simulink model "ADP_USB"  (R2017a)
settings: Solver=ode1  StartTime=0.0  StopTime=30  FixedStep=tau  RelTol=1e-3  EnableMultiTasking=on
InitFcn:
  | ADP_USB_Init
undefined symbols (not defined in the file or in its folder): K, T, tau, wcInit
libraries: simulink x4, simulink_extras x4, quanser_aero x1, quarc_library x1
settings Model: SimulationMode=external  ExtModeTrigDuration=10000  Creator=gjaniak  LastModifiedBy=gjaniak
settings SolverCC: PositivePriorityOrder=on
settings DataIOCC: SaveFormat=Array
settings DebuggingCC: SolverPrmCheckMsg=warning  SFUnexpectedBacktrackingDiag=warning  SFNoUnconditionalDefaultTransitionDiag=warning  SFExecutionAtInitializationDiag=none
settings ModelReferenceCC: PropagateSignalLabelsOutOfModel=off
settings RTWCC: SystemTargetFile=quarc_win64.tlc  TemplateMakefile=quarc_default_tmf  Description=QUARC Win64 Target
settings STFCustomTargetCC: TargetPreCompLibLocation=C:\PROGRA~3\QUARC\lib\2017a\win64\release  TargetLangStandard=C99 (ISO)  ConcurrentExecutionCompliant=on  SystemTargetFile=quarc_win64.tlc
settings GRTTargetCC: TargetPreCompLibLocation=C:\PROGRA~3\QUARC\lib\2017a\win64\release  ParMdlRefBuildCompliant=off  CompOptLevelCompliant=off  CombineOutputUpdateFcns=off  MatFileLogging=off  CPPClassGenCompliant=off  GRTInterface=on  UseToolchainInfoCompliant=off  ExtMode=on  ExtModeMexFile=quarc_comm

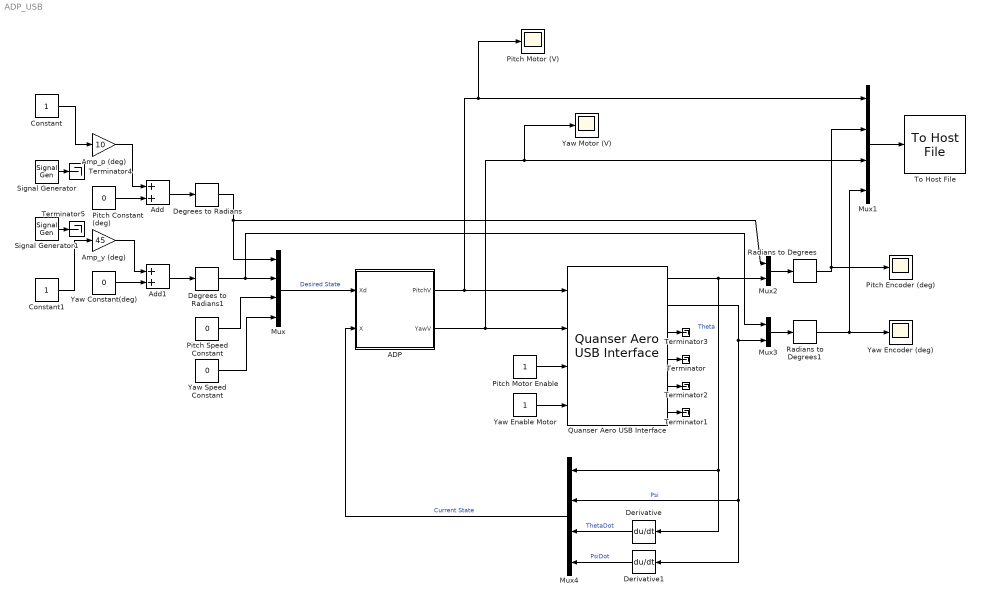
== system ADP_USB ==
  ADP : Subsystem
  Add : Sum
  Add1 : Sum
  Amp_p (deg) : Gain  Gain=10
  Amp_y (deg) : Gain  Gain=45
  Constant : Constant
  Constant1 : Constant
  Degrees to Radians : simulink_extras/Transformations/Degrees to Radians
  Degrees to Radians1 : simulink_extras/Transformations/Degrees to Radians
  Derivative : Derivative
  Derivative1 : Derivative
  Mux : Mux
  Mux1 : Mux
  Mux2 : Mux  Inputs=2
  Mux3 : Mux  Inputs=2
  Mux4 : Mux
  Pitch Constant (deg) : Constant  Value=0
  Pitch Encoder (deg) : Scope
  Pitch Motor (V) : Scope
  Pitch Motor Enable : Constant
  Pitch Speed Constant : Constant  Value=0
  Quanser Aero USB Interface : quanser_aero/Quanser Aero USB Interface
  Radians to Degrees : simulink_extras/Transformations/Radians to Degrees
  Radians to Degrees1 : simulink_extras/Transformations/Radians to Degrees
  Signal Generator : SignalGenerator  WaveForm=square  Frequency=0.1
  Signal Generator1 : SignalGenerator  WaveForm=square  Frequency=0.04
  Terminator{,1..5} (6 alike) : Terminator
  To Host File : quarc_library/Sinks/To Host/To Host File  file_name=ADP_USB_Square.mat  variable_name=ADP_USB_Square  decimation=1  sample_time=-1  file_format=MAT-file v.4  options=No header or footer  append=off  final_file_name=ADP_USB_Square.mat  bitrate=2000000
  Yaw Constant(deg) : Constant  Value=0
  Yaw Enable Motor : Constant
  Yaw Encoder (deg) : Scope
  Yaw Motor (V) : Scope
  Yaw Speed Constant : Constant  Value=0
  wires:
  Yaw Enable Motor/1 -> Quanser Aero USB Interface/4
  Pitch Motor Enable/1 -> Quanser Aero USB Interface/3
  Quanser Aero USB Interface/4 -> Terminator/1
  Quanser Aero USB Interface/6 -> Terminator1/1
  Quanser Aero USB Interface/5 -> Terminator2/1
  Quanser Aero USB Interface/3 -> Terminator3/1
  Pitch Constant (deg)/1 -> Add/2
  Add1/1 -> Degrees to Radians1/1
  Amp_p (deg)/1 -> Add/1
  Yaw Constant(deg)/1 -> Add1/2
  Add/1 -> Degrees to Radians/1
  Amp_y (deg)/1 -> Add1/1
  Degrees to Radians/1 -> Mux2/1, Mux/1
  Degrees to Radians1/1 -> Mux3/1, Mux/2
  Pitch Speed Constant/1 -> Mux/3
  Yaw Speed Constant/1 -> Mux/4
  Quanser Aero USB Interface/1 -> Derivative/1, Mux4/1, Mux2/2  "Theta"
  Quanser Aero USB Interface/2 -> Derivative1/1, Mux4/2, Mux3/2  "Psi"
  Mux/1 -> ADP/1(Xd)  "Desired State"
  Mux1/1 -> To Host File/1
  ADP/1(PitchV) -> Pitch Motor (V)/1, Mux1/1, Quanser Aero USB Interface/1
  ADP/2(YawV) -> Yaw Motor (V)/1, Mux1/3, Quanser Aero USB Interface/2
  Mux3/1 -> Radians to Degrees1/1
  Mux2/1 -> Radians to Degrees/1
  Radians to Degrees/1 -> Pitch Encoder (deg)/1, Mux1/2
  Radians to Degrees1/1 -> Yaw Encoder (deg)/1, Mux1/4
  Derivative/1 -> Mux4/3  "ThetaDot"
  Derivative1/1 -> Mux4/4  "PsiDot"
  Mux4/1 -> ADP/2(X)  "Current State"
  Signal Generator/1 -> Terminator4/1
  Constant/1 -> Amp_p (deg)/1
  Signal Generator1/1 -> Terminator5/1
  Constant1/1 -> Amp_y (deg)/1

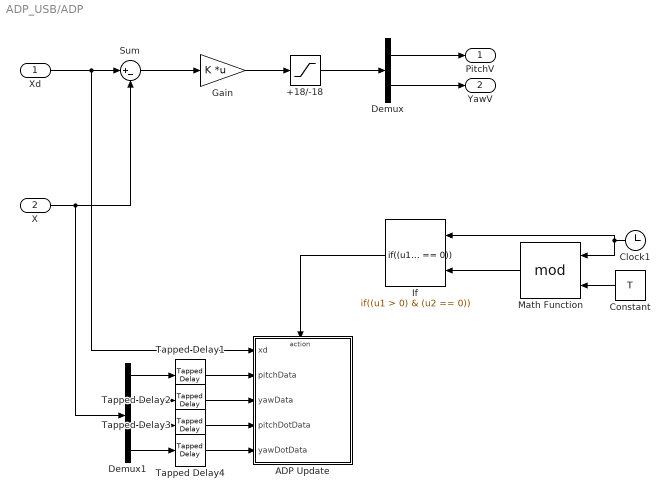
== system ADP_USB/ADP ==
  Xd : Inport
  X : Inport  Port=2
  +18/-18 : Saturate  UpperLimit=18  LowerLimit=-18
  ADP Update : Subsystem  TreatAsAtomicUnit=on
  Clock1 : Clock
  Constant : Constant  Value=T
  Demux : Demux  Outputs=2
  Demux1 : Demux
  Gain : Gain  Gain=K  Multiplication=Matrix(K*u)
  If : If  NumInputs=2  IfExpression=(u1 > 0) & (u2 == 0)  ShowElse=off
  Math Function : Math  Operator=mod  SaturateOnIntegerOverflow=on
  Sum : Sum  Inputs=|+-
  Tapped Delay{1..4} (4 alike) : simulink/Discrete/Tapped Delay  vinit=0.0  samptime=-1  NumDelays=floor(T/tau)  DelayOrder=Oldest  includeCurrent=off
  PitchV : Outport
  YawV : Outport  Port=2
  wires:
  Xd/1 -> ADP Update/1(xd), Sum/1
  Sum/1 -> Gain/1
  Gain/1 -> +18/-18/1
  +18/-18/1 -> Demux/1
  Demux/1 -> PitchV/1
  Demux/2 -> YawV/1
  If/1 -> ADP Update/Action
  Math Function/1 -> If/2
  Constant/1 -> Math Function/2
  Clock1/1 -> If/1, Math Function/1
  X/1 -> Demux1/1, Sum/2
  Demux1/1 -> Tapped Delay1/1
  Tapped Delay1/1 -> ADP Update/2(pitchData)
  Demux1/2 -> Tapped Delay2/1
  Tapped Delay2/1 -> ADP Update/3(yawData)
  Demux1/3 -> Tapped Delay3/1
  Tapped Delay3/1 -> ADP Update/4(pitchDotData)
  Demux1/4 -> Tapped Delay4/1
  Tapped Delay4/1 -> ADP Update/5(yawDotData)

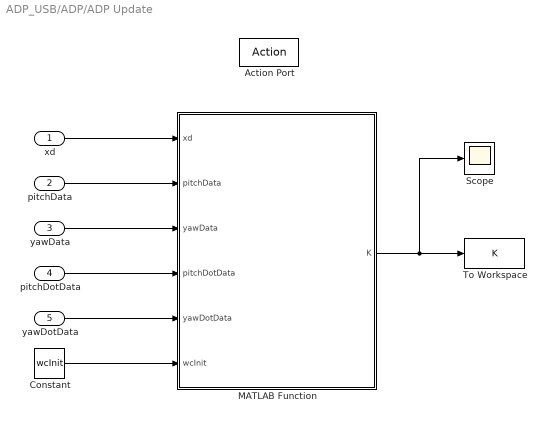
== system ADP_USB/ADP/ADP Update ==
  xd : Inport
  pitchData : Inport  Port=2
  yawData : Inport  Port=3
  pitchDotData : Inport  Port=4
  yawDotData : Inport  Port=5
  Action Port : ActionPort  ActionType=then
  Constant : Constant  Value=wcInit
  MATLAB Function : MATLAB Function  TreatAsAtomicUnit=on
  Scope : Scope
  To Workspace : ToWorkspace  VariableName=K  SampleTime=-1
  wires:
  MATLAB Function/1(K) -> Scope/1, To Workspace/1
  yawData/1 -> MATLAB Function/3(yawData)
  pitchDotData/1 -> MATLAB Function/4(pitchDotData)
  yawDotData/1 -> MATLAB Function/5(yawDotData)
  pitchData/1 -> MATLAB Function/2(pitchData)
  xd/1 -> MATLAB Function/1(xd)
  Constant/1 -> MATLAB Function/6(wcInit)

== matlab function ADP_USB/ADP/ADP Update/MATLAB Function ==
  data: xd input; pitchData input; yawData input; pitchDotData input; yawDotData input; K output; wcInit input
% CRITIC WEIGHT TUNING NEURAL NETWORK
% This function is specific to the helicopter because of the number of
% weights and error model
% THIS FUNCTION CANNOT HAVE ANY ANONYMOUS FUNCTIONS DUE TO THE C CODE
% GENERATION UNSUPPORTING IT
function K = quanserAEROCriticTuning(xd,pitchData,yawData,pitchDotData,yawDotData,wcInit)
    % CREATE THE ERROR VECTOR MATRIX
    % Use the data from the tapped delay blocks to create the error state
    % vector matrix
    e_vec = [pitchData'; yawData'; pitchDotData'; yawDotData'];
    
    % REFERENCE DR. MIAH'S PAPER FOR EQUATION NUMBERS
    % Sampling time [s]
    tau = 0.05;
    
    % COST FUNCTION
    % Q and R matrices used in the cost function
    Q_Mat = diag([270 100 1 1]);
    R_Mat = 0.005*diag([1 1]);
    
    % SYSTEM PARAMETERS SPECIFIC TO THE 2-DOF QUANSER AERO
    A = [0 0 1 0; 0 0 0 1; -1.7442 0 -0.3307 0; 0 0 0 -0.9283];
    B = [0 0; 0 0; -0.0149 0.0414; -0.0751 -0.1295];
    % UNCOMMENT TO USE A STATE-SPACE MODEL THAT IS NOT THE CORRECT ONE DERIVED
    % A = [1 1 1 1; 1 1 1 1; 1 1 1 1; 1 1 1 1];
    % B = [0 0; 0 0; 0.1 0.1; -0.3 -0.3];
    % System dimensions specific for our model
    [n,~] = size(B);
    
    % ERROR MODEL OF THE HELICOPTER
    % gbar and hbar -- EQ 8
    % An anonymous function cannot be used for fbar
    gbar = -B;
    hbar = -A*xd;
    
    % DISCRETE-TIME ERROR MODEL FOR TIME TAU
    % g and h -- EQ 10
    % An anonymous function cannot be used for f
    g = gbar*tau;
    h = hbar*tau;
    
    % COST FUNCTION PARAMETERS
    % The Q matrix cannot be treated as an anonymous function as in the
    % MATLAB simulations
    % Control penalizing matrix in the continuous cost function
    Rbar = R_Mat;
    % The discrete-time cost function will have terms:
    % Right after EQ 11 in paper
    % Control penalizing matrix in the discretized cost function
    R = Rbar*tau;
    
    % NEURAL NETWORK FUNCTIONS
    % These functions cannot be written as anonymous functions as in the
    % MATLAB simulations
    
    % TOLERANCES
    % Convergence tolerance for control policy 
    EpsilonPolicy = 0.1;
    % Convergence tolerance for critic neural network
    EpsilonWcritic = 0.1;
    
    % TRAINING PARAMETERS
    % Number of outer loop iterations
    outerLoopMax = 700;
    % Number of inner loop iterations
    innerLoopMax = 100;
    % Number of equations needed for training, number of sub-intervals
    % Number of training samples
    [~,nbar] = size(e_vec);

    % WEIGHT INITIALIZATION
    % Initialize the weights of the critic neural network to zero
    % Number of rows hard-coded for the helicopter
    WcLast = zeros(14,1);
    
    % LEAST-SQUARES COMPUTATION INITIALIZATION
    % Matrices required for computing least squares weights of the critic 
    % neural networks -- EQ 20
    V = zeros(nbar,1);
    Lambda = zeros(nbar,14);
    
    % Matrix to hold the derivative of the error model during policy
    % updating
    e_k_plus_1 = zeros(n,nbar);
    
    % Product of the least squares matrices must be invertible
    % Logic flag indicating if the critic weights are unsolvable
    % The weights are unsolvable because the least squares matrices have no
    % solution -- not invertible
    diverged = 0;
    
    % OUTER LOOP
    for i = 1:(outerLoopMax-1)
    % Determine if the least squares matrices are invertible
    if diverged == 0
        % For each of the data collection (discrete time index)
        for k = 1:nbar
            % Initialize the optimal inputs to zero 
            uNew = [0; 0];
            % INNER LOOP
            for j = 1:(innerLoopMax-1)
                % Get the updated input value
                uLast = uNew;
                % Update the error model
                % Because of no anonymous functions we have modified f
                % fbar = @(e) A*e;
                % f = @(e) fbar(e)*tau + e;
                e_k_plus_1(:,k) = (A*e_vec(:,k)*tau) + e_vec(:,k) + g*uLast + h;
                % Compute the new optimal inputs
                % Partial derivative of rho with respect to e
                drhode = [1, 0, 0, 0;
                          0, 1, 0, 0;
                          0, 0, 1, 0;
                          0, 0, 0, 1;
                          2*e_vec(1,k), 0, 0, 0;
                          e_vec(2,k), e_vec(1,k), 0, 0;
                          e_vec(3,k), 0, e_vec(1,k), 0;
                          e_vec(4,k), 0, 0, e_vec(1,k);
                          0, 2*e_vec(2,k), 0, 0;
                          0, e_vec(3,k), e_vec(2,k), 0;
                          0, e_vec(4,k), 0, e_vec(2,k);
                          0, 0, 2*e_vec(3,k), 0;
                          0, 0, e_vec(4,k), e_vec(3,k);
                          0, 0, 0, 2*e_vec(4,k)];
                uNew  = -0.5*(R^(-1))*g'*drhode'*WcLast;
                
                % Check convergence of the optimal inputs
                if norm(uNew - uLast) < EpsilonPolicy
                    break;
                end
            end

            % Update the values for the least-squares computation
            % Critic neural network activation functions
            rhoE = [e_vec(1,k); e_vec(2,k); e_vec(3,k); e_vec(4,k);...
                    e_vec(1,k)^2; e_vec(1,k)*e_vec(2,k);...
                    e_vec(1,k)*e_vec(3,k); e_vec(1,k)*e_vec(4,k);...
                    e_vec(2,k)^2; e_vec(2,k)*e_vec(3,k);...
                    e_vec(2,k)*e_vec(4,k); e_vec(3,k)^2;...
                    e_vec(3,k)*e_vec(4,k); e_vec(4,k)^2];
           rhoEK = [e_k_plus_1(1,k); e_k_plus_1(2,k); e_k_plus_1(3,k);...
                    e_k_plus_1(4,k); e_k_plus_1(1,k)^2;...
                    e_k_plus_1(1,k)*e_k_plus_1(2,k);...
                    e_k_plus_1(1,k)*e_k_plus_1(3,k);...
                    e_k_plus_1(1,k)*e_k_plus_1(4,k);...
                    e_k_plus_1(2,k)^2; e_k_plus_1(2,k)*e_k_plus_1(3,k);...
                    e_k_plus_1(2,k)*e_k_plus_1(4,k); e_k_plus_1(3,k)^2;...
                    e_k_plus_1(3,k)*e_k_plus_1(4,k); e_k_plus_1(4,k)^2];
            % State penalizing function in the continuous cost function
            % Qbar = @(e) e'*Q_Mat*e; 
            % State penalizing function in the discretized cost function
            % Q = @(e) Qbar(e)*tau;
            V(k,:) = (e_vec(:,k)'*Q_Mat*e_vec(:,k)*tau) + uNew'*R*uNew + WcLast'*rhoEK;
            Lambda(k,:) = rhoE';
        end
    end

    % Verify the least square solution exists for the critic's weights
    % If the error data is consistent or there is no error, this will not
    % hold, so set the weights to what they were initially before the
    % simulation
    if det(Lambda'*Lambda) == 0
        weights = wcInit;
        break;
    end;

    % Calulcate least squares solution of critic's weights -- EQ 20
    WcNew = (Lambda'*Lambda)^(-1)*Lambda'*V;
    % Make sure the weights did not diverge
    % If the weights diverged, set the weights to what they were initially
    % before the simulation
    if isnan(WcNew)
        weights = wcInit;
        break;
    % Check for convergence of the critic weights
    elseif norm(WcNew - WcLast) < EpsilonWcritic               
        weights = WcNew;
        break;
    % If we reach the last iteration of the loop, just use the last weights
    elseif (i == (outerLoopMax-1))
        weights = WcNew;
    % If all else fails, just set the weights to the initial weights
    else
        weights = wcInit;
    end
    % If the weights did not converge, do another iteration of the loop
    WcLast = WcNew;
    end
    
    % Use the weights to determine the P matrix
    P_Mat = [weights(5) weights(6) weights(7) weights(8);
             weights(6) weights(9) weights(10) weights(11);
             weights(7) weights(10) weights(12) weights(13);
             weights(8) weights(11) weights(13) weights(14)];

    % Find the state-feedback gain EQ
    K = 0.5*(R_Mat^-1)*B'*P_Mat;
end
